simulink model "NUgus"  (R2018a)
settings: Solver=VariableStepAuto  StartTime=0.0  StopTime=inf  RelTol=1e-2
values from neighbouring files (symbols this model uses):
  CM740_acc_bias = 4 * 9.80743    (= 39.22972)    [CM740_init.m]
  CM740_acc_gain = 512 / CM740_acc_centre    [CM740_init.m]
  CM740_gyro_bias = 1600 / 360 * 2 * pi    (= 27.9252680319)    [CM740_init.m]
  CM740_gyro_gain = 512 / CM740_gyro_centre    [CM740_init.m]
  g = 9.8107    [init.m]
  head = [-0.05482228998067195, -0.00010888238321339966, 0.0011712900228573724, 0.41900000000000004]    [comtest.m]
  Kw = 0.9    [init.m]
  model = NUgusKinematics()    [KinematicsTest.m]    (also in Support_Region.m; init.m = NUgusKinematics)
  period = 1.0    (= 1)    [init.m]
  s = mean(abs(present_speed.data))    [RunServoTest.m]
  sample_time = 1/90    (= 0.0111111111111)    [init.m]
  step_height = 0.1    [init.m]
  torso = [0.0050079703254699804, 0.008880921777563762, 0.1021503146237477, 2.5390000000000006]    [comtest.m]
  z0 = 0.45    [init.m]
undefined symbols (not defined in the file or in its folder): sigbuilder_block, X, Y, Z
libraries: sm_lib x206, nesl_utility x82, Contact_Forces_Lib x10
(part 1 of 7)
settings Model: Creator=matt  LastModifiedBy=matt
settings SolverCC: MaxConsecutiveZCs=100  MinimalZcImpactIntegration=on
settings DebuggingCC: UniqueDataStoreMsg=error
settings ModelReferenceCC: ParallelModelReferenceMATLABWorkerInit=Copy Base Workspace  ModelReferenceNumInstancesAllowed=Single  ModelReferenceMinAlgLoopOccurrences=on
settings DiagnosticsConfigSet: SimMechanicsRigidlyBoundBlock=warning
settings ExplorerConfigSet: InternalSimMechanicsExplorerSettings="<ExplorerConfiguration><canonicalview>default</canonicalview><AnimationSetting><BasePlaybackSpeed>1.0</BasePlaybackSpeed><PlaybackSpeedFactor>0.125</PlaybackSpeedFactor></AnimationSetting><TilePanel><TileInfo><Tiles Columns=\"1\" Count=\"1\" Rows=\"1\"><Column Weight=\"1\"/><Row Weight=\"1\"/><Tile Height=\"1\" Width=\"1\" X=\"0\" Y=\"0\"/></Tiles></TileInfo><SceneInfo><SceneViewer><BGColor><R>0.800000011920928955</R><G>0.800000011920928955</G><B>0.800000011920928955</B></BGColor><Camera><DoPerspective>off</DoPerspective><Position><X>0.996097398048217064</X><Y>-0.871904325438711214</Y><Z>0.621451067428618886</Z></Position><Center><X>-0.122665475521987533</X><Y>0.224636309977359006</Y><Z>0.297935636755597033</Z></Center><Up><X>-0.160360573572373266</X><Y>0.125250173842771817</Y><Z>0.97907960881426559</Z></Up><ViewLimDist>1</ViewLimDist><YLim>0.594254607494361209</YLim><XLim>0.353738210919678941</XLim></Camera></SceneViewer></SceneInfo></TilePanel><MechEditorPanel><Cameras/><GfxPanelCameraMap/><VideoCreator><PlaybackSpeedRatio>1.0</PlaybackSpeedRatio><FrameRate>30</FrameRate><VideoFormat>Motion JPEG AVI</VideoFormat><FrameSize>auto</FrameSize></VideoCreator></MechEditorPanel></ExplorerConfiguration>"

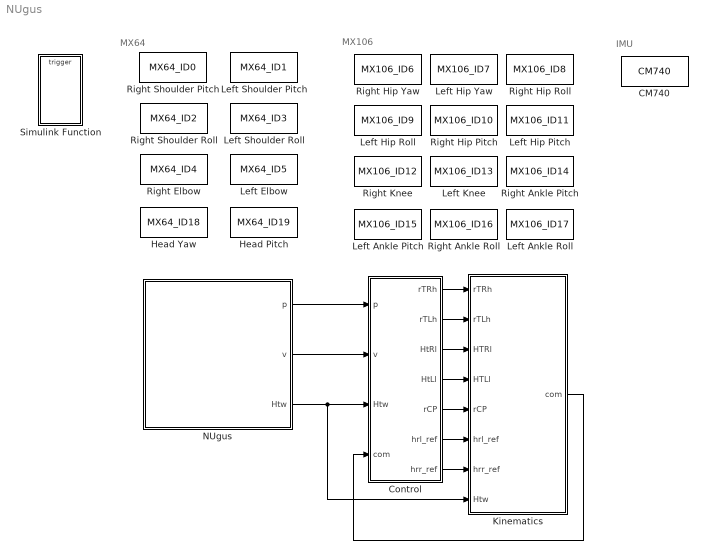
== system NUgus ==
  note: IMU
  note: MX64
  note: MX106
  CM740 : DataStoreMemory  DataStoreName=CM740  ReadBeforeWriteMsg=warning  WriteAfterWriteMsg=warning  WriteAfterReadMsg=warning  InitialValue=CM740_default  VectorParams1D=off  ShowAdditionalParam=off  OutDataTypeStr=Bus: CM740_bus
  Control : Subsystem
  Head Pitch : DataStoreMemory  DataStoreName=MX64_ID19  ReadBeforeWriteMsg=warning  WriteAfterWriteMsg=warning  WriteAfterReadMsg=warning  InitialValue=MX64_default  VectorParams1D=off  ShowAdditionalParam=off  OutDataTypeStr=Bus: MX64_bus
  Head Yaw : DataStoreMemory  DataStoreName=MX64_ID18  ReadBeforeWriteMsg=warning  WriteAfterWriteMsg=warning  WriteAfterReadMsg=warning  InitialValue=MX64_default  VectorParams1D=off  ShowAdditionalParam=off  OutDataTypeStr=Bus: MX64_bus
  Kinematics : Subsystem
  Left Ankle Pitch : DataStoreMemory  DataStoreName=MX106_ID15  ReadBeforeWriteMsg=warning  WriteAfterWriteMsg=warning  WriteAfterReadMsg=warning  InitialValue=MX106_default  VectorParams1D=off  ShowAdditionalParam=off  OutDataTypeStr=Bus: MX106_bus
  Left Ankle Roll : DataStoreMemory  DataStoreName=MX106_ID17  ReadBeforeWriteMsg=warning  WriteAfterWriteMsg=warning  WriteAfterReadMsg=warning  InitialValue=MX106_default  VectorParams1D=off  ShowAdditionalParam=off  OutDataTypeStr=Bus: MX106_bus
  Left Elbow : DataStoreMemory  DataStoreName=MX64_ID5  ReadBeforeWriteMsg=warning  WriteAfterWriteMsg=warning  WriteAfterReadMsg=warning  InitialValue=MX64_default  VectorParams1D=off  ShowAdditionalParam=off  OutDataTypeStr=Bus: MX64_bus
  Left Hip Pitch : DataStoreMemory  DataStoreName=MX106_ID11  ReadBeforeWriteMsg=warning  WriteAfterWriteMsg=warning  WriteAfterReadMsg=warning  InitialValue=MX106_default  VectorParams1D=off  ShowAdditionalParam=off  OutDataTypeStr=Bus: MX106_bus
  Left Hip Roll : DataStoreMemory  DataStoreName=MX106_ID9  ReadBeforeWriteMsg=warning  WriteAfterWriteMsg=warning  WriteAfterReadMsg=warning  InitialValue=MX106_default  VectorParams1D=off  ShowAdditionalParam=off  OutDataTypeStr=Bus: MX106_bus
  Left Hip Yaw : DataStoreMemory  DataStoreName=MX106_ID7  ReadBeforeWriteMsg=warning  WriteAfterWriteMsg=warning  WriteAfterReadMsg=warning  InitialValue=MX106_default  VectorParams1D=off  ShowAdditionalParam=off  OutDataTypeStr=Bus: MX106_bus
  Left Knee : DataStoreMemory  DataStoreName=MX106_ID13  ReadBeforeWriteMsg=warning  WriteAfterWriteMsg=warning  WriteAfterReadMsg=warning  InitialValue=MX106_default  VectorParams1D=off  ShowAdditionalParam=off  OutDataTypeStr=Bus: MX106_bus
  Left Shoulder Pitch : DataStoreMemory  DataStoreName=MX64_ID1  ReadBeforeWriteMsg=warning  WriteAfterWriteMsg=warning  WriteAfterReadMsg=warning  InitialValue=MX64_default  VectorParams1D=off  ShowAdditionalParam=off  OutDataTypeStr=Bus: MX64_bus
  Left Shoulder Roll : DataStoreMemory  DataStoreName=MX64_ID3  ReadBeforeWriteMsg=warning  WriteAfterWriteMsg=warning  WriteAfterReadMsg=warning  InitialValue=MX64_default  VectorParams1D=off  ShowAdditionalParam=off  OutDataTypeStr=Bus: MX64_bus
  NUgus : Subsystem
      mask Display: image('./img/NUgus.png');
  Right Ankle Pitch : DataStoreMemory  DataStoreName=MX106_ID14  ReadBeforeWriteMsg=warning  WriteAfterWriteMsg=warning  WriteAfterReadMsg=warning  InitialValue=MX106_default  VectorParams1D=off  ShowAdditionalParam=off  OutDataTypeStr=Bus: MX106_bus
  Right Ankle Roll : DataStoreMemory  DataStoreName=MX106_ID16  ReadBeforeWriteMsg=warning  WriteAfterWriteMsg=warning  WriteAfterReadMsg=warning  InitialValue=MX106_default  VectorParams1D=off  ShowAdditionalParam=off  OutDataTypeStr=Bus: MX106_bus
  Right Elbow : DataStoreMemory  DataStoreName=MX64_ID4  ReadBeforeWriteMsg=warning  WriteAfterWriteMsg=warning  WriteAfterReadMsg=warning  InitialValue=MX64_default  VectorParams1D=off  ShowAdditionalParam=off  OutDataTypeStr=Bus: MX64_bus
  Right Hip Pitch : DataStoreMemory  DataStoreName=MX106_ID10  ReadBeforeWriteMsg=warning  WriteAfterWriteMsg=warning  WriteAfterReadMsg=warning  InitialValue=MX106_default  VectorParams1D=off  ShowAdditionalParam=off  OutDataTypeStr=Bus: MX106_bus
  Right Hip Roll : DataStoreMemory  DataStoreName=MX106_ID8  ReadBeforeWriteMsg=warning  WriteAfterWriteMsg=warning  WriteAfterReadMsg=warning  InitialValue=MX106_default  VectorParams1D=off  ShowAdditionalParam=off  OutDataTypeStr=Bus: MX106_bus
  Right Hip Yaw : DataStoreMemory  DataStoreName=MX106_ID6  InitialValue=MX106_default  VectorParams1D=off  ShowAdditionalParam=off  OutDataTypeStr=Bus: MX106_bus
  Right Knee : DataStoreMemory  DataStoreName=MX106_ID12  ReadBeforeWriteMsg=warning  WriteAfterWriteMsg=warning  WriteAfterReadMsg=warning  InitialValue=MX106_default  VectorParams1D=off  ShowAdditionalParam=off  OutDataTypeStr=Bus: MX106_bus
  Right Shoulder Pitch : DataStoreMemory  DataStoreName=MX64_ID0  ReadBeforeWriteMsg=warning  WriteAfterWriteMsg=warning  WriteAfterReadMsg=warning  InitialValue=MX64_default  VectorParams1D=off  ShowAdditionalParam=off  OutDataTypeStr=Bus: MX64_bus
  Right Shoulder Roll : DataStoreMemory  DataStoreName=MX64_ID2  ReadBeforeWriteMsg=warning  WriteAfterWriteMsg=warning  WriteAfterReadMsg=warning  InitialValue=MX64_default  VectorParams1D=off  ShowAdditionalParam=off  OutDataTypeStr=Bus: MX64_bus
  Simulink Function : Subsystem  TreatAsAtomicUnit=on
  wires:
  NUgus/1(p) -> Control/1(p)
  NUgus/2(v) -> Control/2(v)
  Control/1(rTRh) -> Kinematics/1(rTRh)
  Control/2(rTLh) -> Kinematics/2(rTLh)
  Control/3(HtRl) -> Kinematics/3(HTRl)
  Control/4(HtLl) -> Kinematics/4(HTLl)
  Control/5(rCP) -> Kinematics/5(rCP)
  NUgus/3(Htw) -> Control/3(Htw), Kinematics/8(Htw)
  Kinematics/1(com) -> Control/4(com)
  Control/6(hrl_ref) -> Kinematics/6(hrl_ref)
  Control/7(hrr_ref) -> Kinematics/7(hrr_ref)

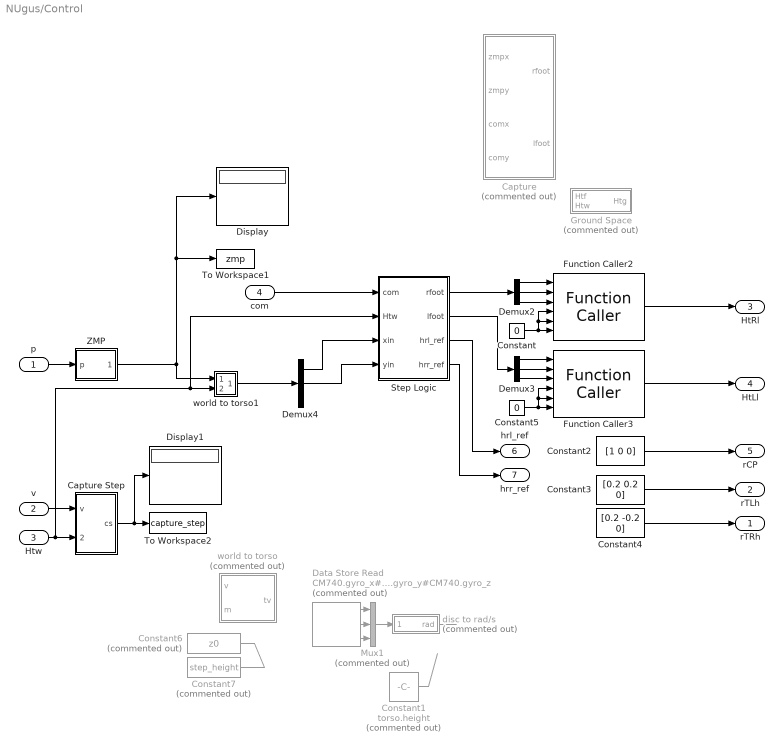
== system NUgus/Control ==
  p : Inport
  v : Inport  Port=2
  Htw : Inport  Port=3
  com : Inport  Port=4
  Capture : Stateflow chart  Commented=on  TreatAsAtomicUnit=on
  Capture Step : Subsystem
  Constant : Constant  Value=0
  Constant1 : Constant  Commented=on  Value=torso.height
  Constant2 : Constant  Value=[1 0 0]
  Constant3 : Constant  Value=[0.2 0.2 0]
  Constant4 : Constant  Value=[0.2 -0.2 0]
  Constant5 : Constant  Value=0
  Constant6 : Constant  Commented=on  Value=z0
  Constant7 : Constant  Commented=on  Value=step_height
  Data Store Read : DataStoreRead  Commented=on  DataStoreName=CM740  SampleTime=1/90  DataStoreElements=CM740.gyro_x#CM740.gyro_y#CM740.gyro_z
  Demux2 : Demux  Outputs=3
  Demux3 : Demux  Outputs=3
  Demux4 : Demux  Outputs=3
  Display : Display
  Display1 : Display
  Function Caller2 : FunctionCaller  FunctionPrototype=H = getTransform(x,y,z,roll,pitch,yaw)
  Function Caller3 : FunctionCaller  FunctionPrototype=H = getTransform(x,y,z,roll,pitch,yaw)
  Ground Space : MATLAB Function  Commented=on  TreatAsAtomicUnit=on
  Mux1 : Mux  Commented=on  Inputs=3
  Step Logic : Stateflow chart  TreatAsAtomicUnit=on
  To Workspace1 : ToWorkspace  VariableName=zmp  SaveFormat=Timeseries  SampleTime=sample_time
  To Workspace2 : ToWorkspace  VariableName=capture_step  SaveFormat=Timeseries  SampleTime=sample_time
  ZMP : Subsystem
  disc to rad/s : Subsystem  Commented=on
  world to torso : Subsystem  Commented=on
  world to torso1 : Subsystem
  rTRh : Outport
  rTLh : Outport  Port=2
  HtRl : Outport  Port=3
  HtLl : Outport  Port=4
  rCP : Outport  Port=5
  hrl_ref : Outport  Port=6
  hrr_ref : Outport  Port=7
  wires:
  Demux2/3 -> Function Caller2/3
  Demux3/3 -> Function Caller3/3
  disc to rad/s/1(rad) -> ?
  Demux3/2 -> Function Caller3/2
  Constant/1 -> Function Caller2/4, Function Caller2/5, Function Caller2/6
  Data Store Read/3 -> Mux1/3
  Step Logic/1(rfoot) -> Demux2/1
  Data Store Read/2 -> Mux1/2
  Mux1/1 -> disc to rad/s/1(disc)
  Demux2/2 -> Function Caller2/2
  Data Store Read/1 -> Mux1/1
  Demux3/1 -> Function Caller3/1
  Demux2/1 -> Function Caller2/1
  Step Logic/2(lfoot) -> Demux3/1
  p/1 -> ZMP/1(p)
  Htw/1 -> Step Logic/2(Htw), world to torso1/2(m), Capture Step/2(Htw)
  Capture Step/1(cs) -> Display1/1, To Workspace2/1
  v/1 -> Capture Step/1(v)
  Constant1/1 -> ?
  Constant2/1 -> rCP/1
  Constant3/1 -> rTLh/1
  Constant4/1 -> rTRh/1
  Constant5/1 -> Function Caller3/4, Function Caller3/5, Function Caller3/6
  Constant6/1 -> ?
  Constant7/1 -> ?
  ZMP/1(zmp) -> world to torso1/1(v), To Workspace1/1, Display/1
  Function Caller3/1 -> HtLl/1
  Function Caller2/1 -> HtRl/1
  Step Logic/3(hrl_ref) -> hrl_ref/1
  Step Logic/4(hrr_ref) -> hrr_ref/1
  Demux4/2 -> Step Logic/4(yin)
  Demux4/1 -> Step Logic/3(xin)
  com/1 -> Step Logic/1(com)
  world to torso1/1(tv) -> Demux4/1

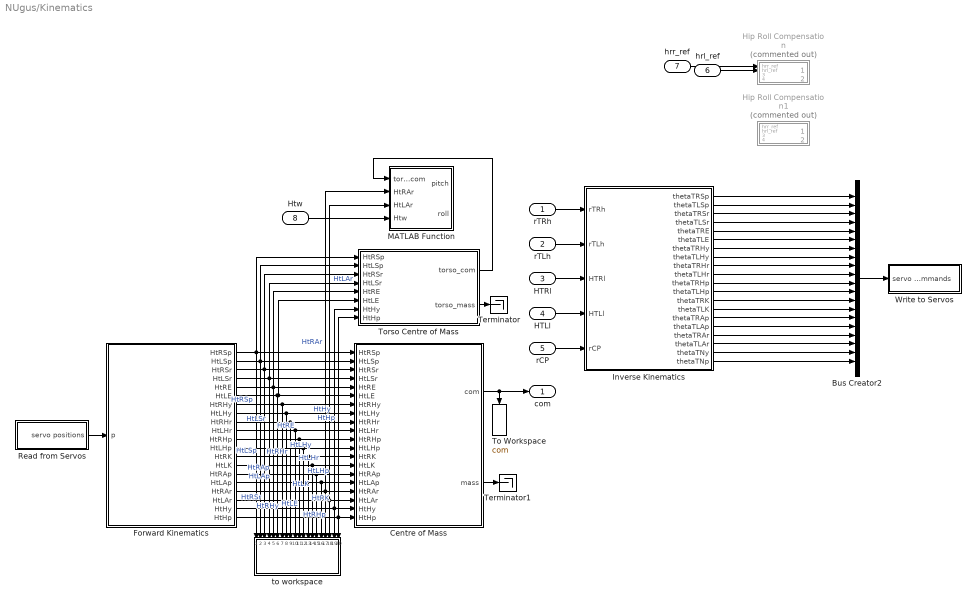
== system NUgus/Kinematics ==
  rTRh : Inport
  rTLh : Inport  Port=2
  HTRl : Inport  Port=3
  HTLl : Inport  Port=4
  rCP : Inport  Port=5
  hrl_ref : Inport  Port=6
  hrr_ref : Inport  Port=7
  Htw : Inport  Port=8
  Bus Creator2 : BusCreator  Inputs=20
  Centre of Mass : Subsystem
  Forward Kinematics : Subsystem
  Hip Roll Compensation : Subsystem  Commented=on
  Hip Roll Compensation1 : Subsystem  Commented=on
  Inverse Kinematics : Subsystem
  MATLAB Function : MATLAB Function  TreatAsAtomicUnit=on  SystemSampleTime=sample_time
  Read from Servos : Subsystem
  Terminator : Terminator
  Terminator1 : Terminator
  To Workspace : ToWorkspace  VariableName=com  SaveFormat=Timeseries  SampleTime=sample_time
  Torso Centre of Mass : Subsystem
  Write to Servos : Subsystem
  to workspace : Subsystem
  com : Outport
  wires:
  Forward Kinematics/10(HtLHr) -> Centre of Mass/10(HtLHr), to workspace/10(HtLHr)  "HtLHr"
  Forward Kinematics/9(HtRHr) -> Centre of Mass/9(HtRHr), to workspace/9(HtRHr)  "HtRHr"
  Forward Kinematics/8(HtLHy) -> Centre of Mass/8(HtLHy), to workspace/8(HtLHy)  "HtLHy"
  Inverse Kinematics/19(thetaTNy) -> Bus Creator2/19
  Forward Kinematics/12(HtLHp) -> Centre of Mass/12(HtLHp), to workspace/12(HtLHp)  "HtLHp"
  Forward Kinematics/15(HtRAp) -> Centre of Mass/15(HtRAp), to workspace/15(HtRAp)  "HtRAp"
  Centre of Mass/1(com) -> com/1, To Workspace/1
  HTLl/1 -> Inverse Kinematics/4(HTLl)
  Forward Kinematics/11(HtRHp) -> Centre of Mass/11(HtRHp), to workspace/11(HtRHp)  "HtRHp"
  Forward Kinematics/4(HtLSr) -> Torso Centre of Mass/4(HtLSr), Centre of Mass/4(HtLSr), to workspace/4(HtLSr)  "HtLSr"
  Inverse Kinematics/5(thetaTRE) -> Bus Creator2/5
  Forward Kinematics/18(HtLAr) -> Centre of Mass/18(HtLAr), MATLAB Function/3(HtLAr), to workspace/18(HtLAr)  "HtLAr"
  rTRh/1 -> Inverse Kinematics/1(rTRh)
  Inverse Kinematics/6(thetaTLE) -> Bus Creator2/6
  Forward Kinematics/6(HtLE) -> Torso Centre of Mass/6(HtLE), Centre of Mass/6(HtLE), to workspace/6(HtLE)  "HtLE"
  Forward Kinematics/14(HtLK) -> Centre of Mass/14(HtLK), to workspace/14(HtLK)  "HtLK"
  Forward Kinematics/13(HtRK) -> Centre of Mass/13(HtRK), to workspace/13(HtRK)  "HtRK"
  Forward Kinematics/3(HtRSr) -> Torso Centre of Mass/3(HtRSr), Centre of Mass/3(HtRSr), to workspace/3(HtRSr)  "HtRSr"
  Inverse Kinematics/14(thetaTLK) -> Bus Creator2/14
  Inverse Kinematics/7(thetaTRHy) -> Bus Creator2/7
  Forward Kinematics/2(HtLSp) -> Torso Centre of Mass/2(HtLSp), Centre of Mass/2(HtLSp), to workspace/2(HtLSp)  "HtLSp"
  Forward Kinematics/7(HtRHy) -> Centre of Mass/7(HtRHy), to workspace/7(HtRHy)  "HtRHy"
  Forward Kinematics/5(HtRE) -> Torso Centre of Mass/5(HtRE), Centre of Mass/5(HtRE), to workspace/5(HtRE)  "HtRE"
  Forward Kinematics/20(HtHp) -> to workspace/20(HtHp), Torso Centre of Mass/8(HtHp), Centre of Mass/20(HtHp)  "HtHp"
  Inverse Kinematics/1(thetaTRSp) -> Bus Creator2/1
  Inverse Kinematics/3(thetaTRSr) -> Bus Creator2/3
  Inverse Kinematics/13(thetaTRK) -> Bus Creator2/13
  Forward Kinematics/16(HtLAp) -> Centre of Mass/16(HtLAp), to workspace/16(HtLAp)  "HtLAp"
  Forward Kinematics/19(HtHy) -> to workspace/19(HtHy), Torso Centre of Mass/7(HtHy), Centre of Mass/19(HtHy)  "HtHy"
  Read from Servos/1(servo positions) -> Forward Kinematics/1(p)
  rTLh/1 -> Inverse Kinematics/2(rTLh)
  Bus Creator2/1 -> Write to Servos/1(servo commands)
  Forward Kinematics/1(HtRSp) -> Torso Centre of Mass/1(HtRSp), Centre of Mass/1(HtRSp), to workspace/1(HtRSp)  "HtRSp"
  Inverse Kinematics/2(thetaTLSp) -> Bus Creator2/2
  Inverse Kinematics/20(thetaTNp) -> Bus Creator2/20
  Inverse Kinematics/4(thetaTLSr) -> Bus Creator2/4
  Forward Kinematics/17(HtRAr) -> to workspace/17(HtRAr), MATLAB Function/2(HtRAr), Centre of Mass/17(HtRAr)  "HtRAr"
  HTRl/1 -> Inverse Kinematics/3(HTRl)
  rCP/1 -> Inverse Kinematics/5(rCP)
  Torso Centre of Mass/2(torso_mass) -> Terminator/1
  Htw/1 -> MATLAB Function/4(Htw)
  Torso Centre of Mass/1(torso_com) -> MATLAB Function/1(torso_com)
  Inverse Kinematics/16(thetaTLAp) -> Bus Creator2/16
  Inverse Kinematics/15(thetaTRAp) -> Bus Creator2/15
  Inverse Kinematics/11(thetaTRHp) -> Bus Creator2/11
  Inverse Kinematics/12(thetaTLHp) -> Bus Creator2/12
  Inverse Kinematics/17(thetaTRAr) -> Bus Creator2/17
  Inverse Kinematics/18(thetaTLAr) -> Bus Creator2/18
  Inverse Kinematics/8(thetaTLHy) -> Bus Creator2/8
  Centre of Mass/2(mass) -> Terminator1/1
  hrl_ref/1 -> Hip Roll Compensation/2(hrl_ref)
  hrr_ref/1 -> Hip Roll Compensation/1("hrr_ref ")
  Inverse Kinematics/9(thetaTRHr) -> Bus Creator2/9
  Inverse Kinematics/10(thetaTLHr) -> Bus Creator2/10

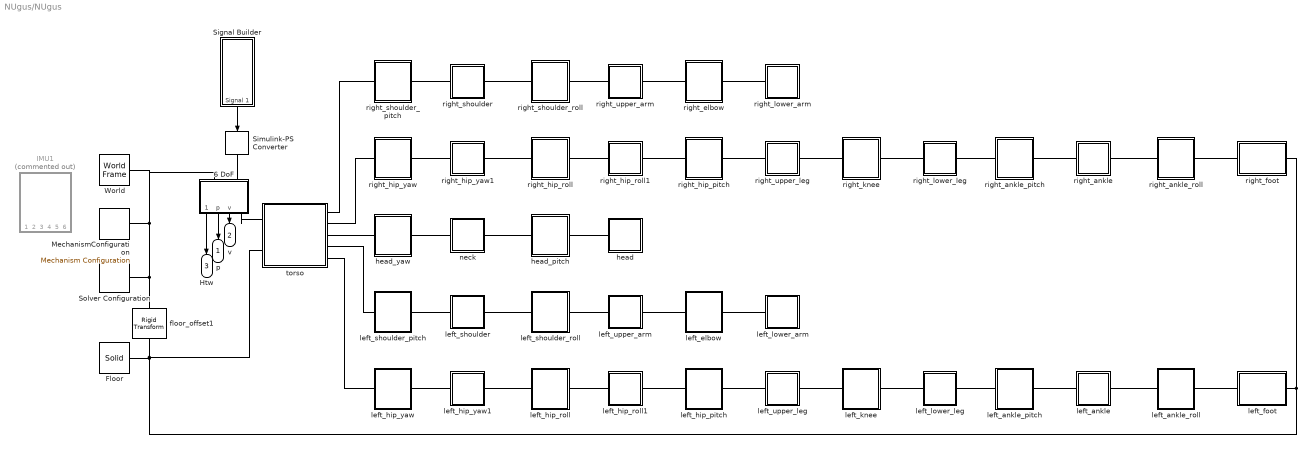
== system NUgus/NUgus ==
  6 DoF : Subsystem
  Floor : sm_lib/Body Elements/Solid  InertiaType=CalculateFromGeometry  Mass=1  MassUnits=kg  CenterOfMass=[0 0 0]  CenterOfMassUnits=m  MomentsOfInertia=[1 1 1]  MomentsOfInertiaUnits=kg*m^2  ProductsOfInertia=[0 0 0]  ProductsOfInertiaUnits=kg*m^2  DensityBased=on  Density=1000  DensityUnits=kg/m^3  DoExposeReferenceFrame=on  SerializedFrames=<Frames/>  GraphicType=FromGeometry  MarkerShape=Frame  MarkerSize=10  GraphicVisPropType=SimpleVisualProperties  GraphicDiffuseColor=[0.972549 0.972549 0.972549]  GraphicSpecularColor=[0.3 0.3 0.3 1.0]  GraphicAmbientColor=[0.20 0.20 0.20 1.0]  GraphicEmissiveColor=[0.0 0.0 0.0 1.0]  GraphicShininess=30  GraphicOpacity=0.6  GeometryShape=Brick  RectangleSize=[1 1]  RectangleSizeUnits=m  BrickDimensions=[floor.length floor.width floor.depth]  BrickDimensionUnits=m  CylinderRadius=1  CylinderRadiusUnits=m  CylinderLength=1  CylinderLengthUnits=m  SphereRadius=1  SphereRadiusUnits=m  EllipsoidRadii=[1 1 1]  EllipsoidRadiiUnits=m  ExtrusionCrossSection=[1 1; -1 1; -1 -1; 1 -1]  ExtrusionCrossSectionUnits=m  ExtrusionLength=1  ExtrusionLengthUnits=m  PolygonNumSides=3  PolygonOuterRadius=1  PolygonOuterRadiusUnits=m  ExtGeomFileType=STEP  ExtGeomFileUnits=m  RevolutionCrossSection=[1 1; 1 -1; 2 -1; 2 1]  RevolutionCrossSectionUnits=m  RevolutionExtent=Full  RevolutionAngle=180  RevolutionAngleUnits=deg
  IMU1 : Subsystem  Commented=on
  MechanismConfiguration : sm_lib/Utilities/Mechanism Configuration  UniformGravity=Constant  GravityVector=[0 0 -9.80665]  GravityUnits=m/s^2  LinearizationDelta=0.001
  Signal Builder : Subsystem  Tag=STV Subsys  LoadFcn=sigbuilder_block('load');  StartFcn=sigbuilder_block('start');  StopFcn=sigbuilder_block('stop');  ClipboardFcn=sigbuilder_block('clipboard');  mask(Sigbuilder block){tuvar=[0:10]}
      mask help: Simulink:masks:SigbuilderBlock_MD
      mask init:
      | if ~strcmp(get_param(bdroot(gcbh),'SimulationStatus'),'stopped') tuvar = sigbuilder_block('maskInit'); end
      settings: CopyFcn=sigbuilder_block('copy');  DeleteFcn=sigbuilder_block('delete');  ModelCloseFcn=sigbuilder_block('modelClose');  PreSaveFcn=sigbuilder_block('preSave');  PauseFcn=sigbuilder_block('pause');  ContinueFcn=sigbuilder_block('continue');  NameChangeFcn=sigbuilder_block('namechange');  OpenFcn=sigbuilder_block('open',[1006.5 174.75 565.5 399.75 ]);  CloseFcn=sigbuilder_block('close');
      mask Display: plot(0, 0, 100, 100,[2, 2, 32, 32, 2], [68, 8, 8, 68, 68],[32, 2], [38, 38], [32, 19, 2],[53, 60, 44], [32, 17, 17, 2],[16, 16, 31, 31]);txt = getActiveGroup(gcbh);text(2, 100, txt,'verticalAlignment', 'top');
  Simulink-PS Converter : nesl_utility/Simulink-PS Converter  PhysicalDomain=network_engine_domain  SubClassName=ps_input  LeftPortType=input  RightPortType=output  PseudoPeriodic=off  Frequencies=[]  NoiseDistribution=none  NoiseParameters=[]  Unit=N  AffineConversion=off  FilteringAndDerivatives=provide  SimscapeFilterOrder=1  InputFilterTimeConstant=0.001  UdotUserProvided=0
  Solver Configuration : nesl_utility/Solver Configuration  PhysicalDomain=network_engine_domain  SubClassName=solver  LeftPortType=input  RightPortType=generic  Tones=[]  Harmonics=[]  SimulateNoise=off  Profile=off  UseLocalSampling=off  EnableSwitchedLinearOptims=on  FrequencyDomain=off  UseCCode=off  RelTol=0.001  AbsTol=1e-06  MinStep=1e-09  ToWorkspace=off  RevertToSquareIcSolve=off  NumHomotopyIterations=100  PhasorMode=off  PhasorModeNumHarmonics=1  DoDC=off  ResidualTolerance=1e-03  UseLocalSolver=off  LocalSolverChoice=NE_BACKWARD_EULER_ADVANCER  LocalSolverSampleTime=0.001  DoFixedCost=off  MaxNonlinIter=3  MaxModeIter=2  LinearAlgebra=Sparse  EquationFormulation=NE_TIME_EF  DelaysMemoryBudget=1024  AutomaticFiltering=on  FilteringTimeConstant=0.001
  World : sm_lib/Frames and Transforms/World Frame
  floor_offset1 : sm_lib/Frames and Transforms/Rigid Transform  TranslationMethod=Cartesian  TranslationStandardOffset=0  TranslationLengthUnit=m  TranslationStandardAxis=+Z  TranslationCartesianOffset=[0 0 -floor.depth/2]  TranslationROffset=0  TranslationROffsetUnits=m  TranslationZOffset=0  TranslationZOffsetUnits=m  TranslationThetaOffset=0  TranslationThetaOffsetUnits=deg  RotationMethod=None  RotationAngleUnits=deg  RotationStandardAxis=+Z  RotationAngle=0.0  RotationArbitraryAxis=[0 0 1]  FollAlignAxisA=+X  BaseAlignAxisA=+Y  FollAlignAxisB=+Y  BaseAlignAxisB=+Z  RotationSequenceAxes=FollowerAxes  RotationSequence=XYX  RotationSequenceAngles=[0 0 0]  RotationSequenceAnglesUnits=deg  RotationMatrix=[1 0 0; 0 1 0; 0 0 1]
  head : Subsystem
  head_pitch : Subsystem
      mask Display: image('./img/MX64.png');
  head_yaw : Subsystem
      mask Display: image('./img/MX64.png');
  left_ankle : Subsystem
  left_ankle_pitch : Subsystem
      mask Display: image('./img/MX106.png');
  left_ankle_roll : Subsystem
      mask Display: image('./img/MX106.png');
  left_elbow : Subsystem
      mask Display: image('./img/MX64.png');
  left_foot : Subsystem
  left_hip_pitch : Subsystem
      mask Display: image('./img/MX106.png');
  left_hip_roll : Subsystem
      mask Display: image('./img/MX106.png');
  left_hip_roll1 : Subsystem
  left_hip_yaw : Subsystem
      mask Display: image('./img/MX106.png');
  left_hip_yaw1 : Subsystem
  left_knee : Subsystem
      mask Display: image('./img/MX106.png');
  left_lower_arm : Subsystem
  left_lower_leg : Subsystem
  left_shoulder : Subsystem
  left_shoulder_pitch : Subsystem
      mask Display: image('./img/MX64.png');
  left_shoulder_roll : Subsystem
      mask Display: image('./img/MX64.png');
  left_upper_arm : Subsystem
  left_upper_leg : Subsystem
  neck : Subsystem
  right_ankle : Subsystem
  right_ankle_pitch : Subsystem
      mask Display: image('./img/MX106.png');
  right_ankle_roll : Subsystem
      mask Display: image('./img/MX106.png');
  right_elbow : Subsystem
      mask Display: image('./img/MX64.png');
  right_foot : Subsystem
  right_hip_pitch : Subsystem
      mask Display: image('./img/MX106.png');
  right_hip_roll : Subsystem
      mask Display: image('./img/MX106.png');
  right_hip_roll1 : Subsystem
  right_hip_yaw : Subsystem
      mask Display: image('./img/MX106.png');
  right_hip_yaw1 : Subsystem
  right_knee : Subsystem
      mask Display: image('./img/MX106.png');
  right_lower_arm : Subsystem
  right_lower_leg : Subsystem
  right_shoulder : Subsystem
  right_shoulder_pitch : Subsystem
      mask Display: image('./img/MX64.png');
  right_shoulder_roll : Subsystem
      mask Display: image('./img/MX64.png');
  right_upper_arm : Subsystem
  right_upper_leg : Subsystem
  torso : Subsystem
  p : Outport
  v : Outport  Port=2
  Htw : Outport  Port=3
  wires:
  Signal Builder/1(Signal 1) -> Simulink-PS Converter/1
  6 DoF/2(p) -> p/1
  6 DoF/3(v) -> v/1
  6 DoF/1(Htw) -> Htw/1
  connections:
  right_ankle_roll/LConn1 -- right_ankle/RConn1
  left_elbow/RConn1 -- left_lower_arm/LConn1
  left_knee/RConn1 -- left_lower_leg/LConn1
  left_hip_roll/LConn1 -- left_hip_yaw1/RConn1
  left_hip_yaw/RConn1 -- left_hip_yaw1/LConn1
  torso/RConn3 -- head_yaw/LConn1
  right_shoulder_roll/LConn1 -- right_shoulder/RConn1
  right_hip_pitch/LConn1 -- right_hip_roll1/RConn1
  right_hip_yaw1/RConn1 -- right_hip_roll/LConn1
  head_pitch/LConn1 -- neck/RConn1
  right_lower_arm/LConn1 -- right_elbow/RConn1
  head/LConn1 -- head_pitch/RConn1
  left_shoulder/RConn1 -- left_shoulder_roll/LConn1
  left_hip_pitch/RConn1 -- left_upper_leg/LConn1
  left_foot/LConn1 -- left_ankle_roll/RConn1
  torso/RConn1 -- right_shoulder_pitch/LConn1
  right_hip_pitch/RConn1 -- right_upper_leg/LConn1
  right_hip_yaw/LConn1 -- torso/RConn2
  left_shoulder_pitch/LConn1 -- torso/RConn4
  left_ankle_pitch/RConn1 -- left_ankle/LConn1
  left_ankle_pitch/LConn1 -- left_lower_leg/RConn1
  left_knee/LConn1 -- left_upper_leg/RConn1
  left_hip_roll/RConn1 -- left_hip_roll1/LConn1
  left_upper_arm/LConn1 -- left_shoulder_roll/RConn1
  left_shoulder_pitch/RConn1 -- left_shoulder/LConn1
  left_ankle_roll/LConn1 -- left_ankle/RConn1
  right_ankle_pitch/RConn1 -- right_ankle/LConn1
  right_ankle_pitch/LConn1 -- right_lower_leg/RConn1
  neck/LConn1 -- head_yaw/RConn1
  right_knee/RConn1 -- right_lower_leg/LConn1
  right_ankle_roll/RConn1 -- right_foot/LConn1
  right_knee/LConn1 -- right_upper_leg/RConn1
  right_hip_roll1/LConn1 -- right_hip_roll/RConn1
  right_shoulder_pitch/RConn1 -- right_shoulder/LConn1
  right_elbow/LConn1 -- right_upper_arm/RConn1
  right_hip_yaw/RConn1 -- right_hip_yaw1/LConn1
  left_elbow/LConn1 -- left_upper_arm/RConn1
  left_hip_roll1/RConn1 -- left_hip_pitch/LConn1
  torso/RConn5 -- left_hip_yaw/LConn1
  right_shoulder_roll/RConn1 -- right_upper_arm/LConn1
  left_foot/RConn1 -- torso/LConn2 -- floor_offset1/RConn1 -- Floor/RConn1 -- right_foot/RConn1
  6 DoF/RConn1 -- torso/LConn1
  MechanismConfiguration/RConn1 -- 6 DoF/LConn1 -- World/RConn1 -- floor_offset1/LConn1 -- Solver Configuration/RConn1
  Simulink-PS Converter/RConn1 -- 6 DoF/LConn2

== system NUgus/Simulink Function ==
  getTransform : TriggerPort  TriggerType=function-call  IsSimulinkFunction=on  FunctionName=getTransform  FunctionVisibility=scoped  VariantControl=(inherit)
  MATLAB Function : MATLAB Function  TreatAsAtomicUnit=on
  x : ArgIn  DisableCoverage=on  ArgumentName=x
  y~ : ArgIn  Port=2  ArgumentName=y
  z : ArgIn  Port=3  ArgumentName=z
  roll : ArgIn  Port=4  ArgumentName=roll
  pitch : ArgIn  Port=5  ArgumentName=pitch
  yaw : ArgIn  Port=6  ArgumentName=yaw
  H : ArgOut  DisableCoverage=on  PortDimensions=[4 4]  ArgumentName=H
  wires:
  x/1 -> MATLAB Function/1(x)
  y~/1 -> MATLAB Function/2(y)
  z/1 -> MATLAB Function/3(z)
  roll/1 -> MATLAB Function/4(roll)
  pitch/1 -> MATLAB Function/5(pitch)
  yaw/1 -> MATLAB Function/6(yaw)
  MATLAB Function/1(H) -> H/1

== system NUgus/Control/Capture Step ==
  v : Inport
  Htw : Inport  Port=2
  Gain : Gain  Gain=sqrt(torso.height/g)
  Matrix Multiply : Product  Multiplication=Matrix(*)
  Subsystem3 : Subsystem
  Subsystem4 : Subsystem
  cs : Outport
  wires:
  Matrix Multiply/1 -> Subsystem4/1(v4)
  Gain/1 -> Subsystem3/1(v3)
  Subsystem4/1(v3) -> cs/1
  v/1 -> Gain/1
  Subsystem3/1(v4) -> Matrix Multiply/2
  Htw/1 -> Matrix Multiply/1

== system NUgus/Control/ZMP ==
  note: zmp z = 0
  note: h = p com,z / g
  note: zmp = p com - ha com
  note: 3D LIPM ZMP Model
  p : Inport
  Add : Sum  Inputs=-+
  Data Store Read : DataStoreRead  DataStoreName=CM740  SampleTime=1/90  DataStoreElements=CM740.acc_x#CM740.acc_y#CM740.acc_z
  Demux : Demux  Outputs=3
  Multiply1 : Product
  Mux : Mux  Inputs=3
  Mux2 : Mux  Inputs=3
  h : Gain  Gain=1/g
  to real : Subsystem
  zmp : Outport
  wires:
  p/1 -> Demux/1
  to real/1(continuous) -> Multiply1/1
  Add/1 -> zmp/1
  Multiply1/1 -> Add/1
  h/1 -> Multiply1/2
  Demux/3 -> Mux2/3, h/1
  Demux/2 -> Mux2/2
  Demux/1 -> Mux2/1
  Mux2/1 -> Add/2
  Data Store Read/2 -> Mux/2
  Data Store Read/1 -> Mux/1
  Data Store Read/3 -> Mux/3
  Mux/1 -> to real/1(discrete)

== system NUgus/Control/disc to rad//s ==
  disc : Inport
  Add1 : Sum  Inputs=+-
  Constant4 : Constant  Value=512
  Gain : Gain  Gain=(500*pi)/(180*512)  OutDataTypeStr=double
  rad : Outport
  wires:
  disc/1 -> Add1/1
  Gain/1 -> rad/1
  Add1/1 -> Gain/1
  Constant4/1 -> Add1/2

== system NUgus/Control/world to torso ==
  v : Inport
  m : Inport  Port=2
  Matrix Multiply : Product  Multiplication=Matrix(*)
  Subsystem3 : Subsystem
  Subsystem4 : Subsystem
  tv : Outport
  wires:
  v/1 -> Subsystem3/1(v3)
  Matrix Multiply/1 -> Subsystem4/1(v4)
  m/1 -> Matrix Multiply/1
  Subsystem4/1(v3) -> tv/1
  Subsystem3/1(v4) -> Matrix Multiply/2

== system NUgus/Control/world to torso1 ==
  v : Inport
  m : Inport  Port=2
  Matrix Multiply : Product  Multiplication=Matrix(*)
  Subsystem3 : Subsystem
  Subsystem4 : Subsystem
  tv : Outport
  wires:
  v/1 -> Subsystem3/1(v3)
  Matrix Multiply/1 -> Subsystem4/1(v4)
  m/1 -> Matrix Multiply/1
  Subsystem4/1(v3) -> tv/1
  Subsystem3/1(v4) -> Matrix Multiply/2

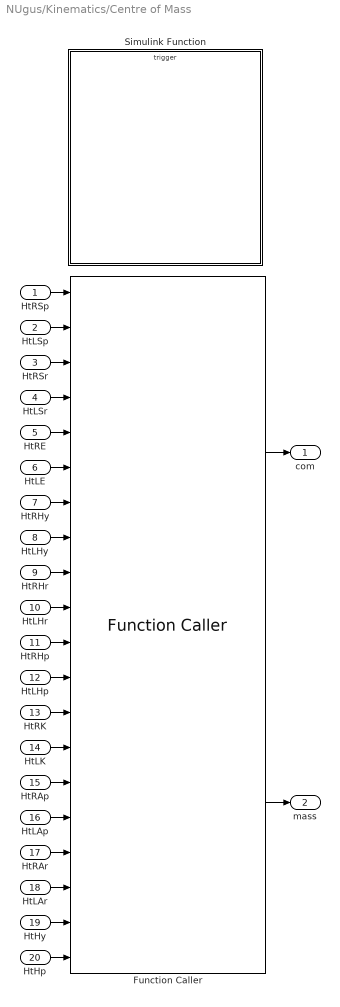
== system NUgus/Kinematics/Centre of Mass ==
  HtRSp : Inport
  HtLSp : Inport  Port=2
  HtRSr : Inport  Port=3
  HtLSr : Inport  Port=4
  HtRE : Inport  Port=5
  HtLE : Inport  Port=6
  HtRHy : Inport  Port=7
  HtLHy : Inport  Port=8
  HtRHr : Inport  Port=9
  HtLHr : Inport  Port=10
  HtRHp : Inport  Port=11
  HtLHp : Inport  Port=12
  HtRK : Inport  Port=13
  HtLK : Inport  Port=14
  HtRAp : Inport  Port=15
  HtLAp : Inport  Port=16
  HtRAr : Inport  Port=17
  HtLAr : Inport  Port=18
  HtHy : Inport  Port=19
  HtHp : Inport  Port=20
  Function Caller : FunctionCaller  FunctionPrototype=[com,mass] = COM(HtRSp,HtLSp,HtRSr,HtLSr,HtRE,HtLE,HtRHy,HtLHy,HtRHr,HtLHr,HtRHp,HtLHp,HtRK,HtLK,HtRAp,HtLAp,HtRAr,HtLAr,HtHy,HtHp)
  Simulink Function : Subsystem  TreatAsAtomicUnit=on
  com : Outport
  mass : Outport  Port=2
  wires:
  HtRK/1 -> Function Caller/13
  HtRHp/1 -> Function Caller/11
  HtHy/1 -> Function Caller/19
  HtLHp/1 -> Function Caller/12
  HtRHr/1 -> Function Caller/9
  HtRE/1 -> Function Caller/5
  HtRHy/1 -> Function Caller/7
  HtRAr/1 -> Function Caller/17
  HtLE/1 -> Function Caller/6
  HtRAp/1 -> Function Caller/15
  HtLHr/1 -> Function Caller/10
  HtLAp/1 -> Function Caller/16
  HtRSr/1 -> Function Caller/3
  HtRSp/1 -> Function Caller/1
  Function Caller/1 -> com/1
  HtLHy/1 -> Function Caller/8
  HtLAr/1 -> Function Caller/18
  HtLK/1 -> Function Caller/14
  HtLSr/1 -> Function Caller/4
  HtLSp/1 -> Function Caller/2
  HtHp/1 -> Function Caller/20
  Function Caller/2 -> mass/1

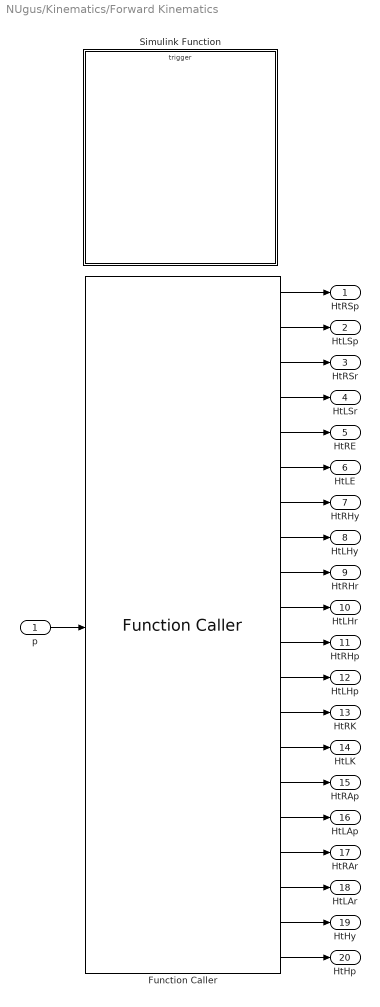
== system NUgus/Kinematics/Forward Kinematics ==
  p : Inport
  Function Caller : FunctionCaller  FunctionPrototype=[HtRSp,HtLSp,HtRSr,HtLSr,HtRE,HtLE,HtRHy,HtLHy,HtRHr,HtLHr,HtRHp,HtLHp,HtRK,HtLK,HtRAp,HtLAp,HtRAr,HtLAr,HtHy,HtHp] = FK(p)  InputArgumentSpecifications=double([1 1 1 1 1 1 1 1 1 1 1 1 1 1 1 1 1 1 1 1])
  Simulink Function : Subsystem  TreatAsAtomicUnit=on
  HtRSp : Outport
  HtLSp : Outport  Port=2
  HtRSr : Outport  Port=3
  HtLSr : Outport  Port=4
  HtRE : Outport  Port=5
  HtLE : Outport  Port=6
  HtRHy : Outport  Port=7
  HtLHy : Outport  Port=8
  HtRHr : Outport  Port=9
  HtLHr : Outport  Port=10
  HtRHp : Outport  Port=11
  HtLHp : Outport  Port=12
  HtRK : Outport  Port=13
  HtLK : Outport  Port=14
  HtRAp : Outport  Port=15
  HtLAp : Outport  Port=16
  HtRAr : Outport  Port=17
  HtLAr : Outport  Port=18
  HtHy : Outport  Port=19
  HtHp : Outport  Port=20
  wires:
  Function Caller/2 -> HtLSp/1
  Function Caller/1 -> HtRSp/1
  Function Caller/3 -> HtRSr/1
  Function Caller/4 -> HtLSr/1
  Function Caller/5 -> HtRE/1
  Function Caller/6 -> HtLE/1
  Function Caller/7 -> HtRHy/1
  Function Caller/8 -> HtLHy/1
  Function Caller/9 -> HtRHr/1
  Function Caller/10 -> HtLHr/1
  Function Caller/11 -> HtRHp/1
  Function Caller/12 -> HtLHp/1
  Function Caller/13 -> HtRK/1
  Function Caller/14 -> HtLK/1
  Function Caller/15 -> HtRAp/1
  Function Caller/16 -> HtLAp/1
  Function Caller/17 -> HtRAr/1
  Function Caller/18 -> HtLAr/1
  Function Caller/19 -> HtHy/1
  Function Caller/20 -> HtHp/1
  p/1 -> Function Caller/1

== system NUgus/Kinematics/Hip Roll Compensation ==
  "hrr_ref " : Inport
  hrl_ref : Inport  Port=2
  theta_ref1 : Inport  Port=3
  theta_ref2 : Inport  Port=4
  Data Store Read : DataStoreRead  Commented=on  DataStoreName=CM740  SampleTime=sample_time  DataStoreElements=CM740.gyro_x
  Inject Control Signal : Subsystem
  Scope : Scope  NumInputPorts=2
  disc to rad/s : Subsystem  Commented=on
  theta_p1 : Outport
  theta_p2 : Outport  Port=2
  wires:
  theta_ref1/1 -> Scope/1, Inject Control Signal/3(theta ref1)
  theta_ref2/1 -> Inject Control Signal/4(theta ref2)
  Data Store Read/1 -> disc to rad/s/1(disc)
  Inject Control Signal/2(theta p2) -> theta_p2/1
  Inject Control Signal/1(theta p1) -> theta_p1/1, Scope/2
  "hrr_ref "/1 -> Inject Control Signal/1(hrr_ref)
  hrl_ref/1 -> Inject Control Signal/2(hrl_ref)

== system NUgus/Kinematics/Hip Roll Compensation1 ==
  "hrr_ref " : Inport
  hrl_ref : Inport  Port=2
  theta_ref1 : Inport  Port=3
  theta_ref2 : Inport  Port=4
  Data Store Read : DataStoreRead  Commented=on  DataStoreName=CM740  SampleTime=sample_time  DataStoreElements=CM740.gyro_x
  Inject Control Signal : Subsystem
  Scope : Scope  NumInputPorts=2
  disc to rad/s : Subsystem  Commented=on
  theta_p1 : Outport
  theta_p2 : Outport  Port=2
  wires:
  theta_ref1/1 -> Scope/1, Inject Control Signal/3(theta ref1)
  theta_ref2/1 -> Inject Control Signal/4(theta ref2)
  Data Store Read/1 -> disc to rad/s/1(disc)
  Inject Control Signal/2(theta p2) -> theta_p2/1
  Inject Control Signal/1(theta p1) -> theta_p1/1, Scope/2
  "hrr_ref "/1 -> Inject Control Signal/1(hrr_ref)
  hrl_ref/1 -> Inject Control Signal/2(hrl_ref)

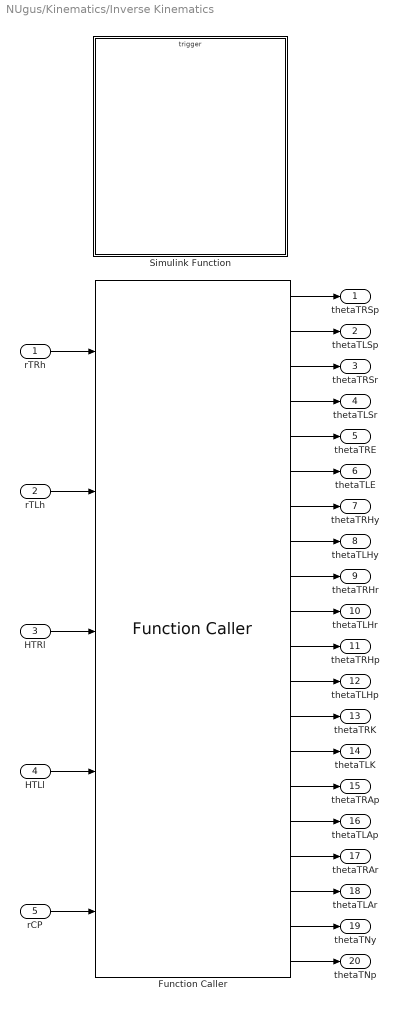
== system NUgus/Kinematics/Inverse Kinematics ==
  rTRh : Inport
  rTLh : Inport  Port=2
  HTRl : Inport  Port=3
  HTLl : Inport  Port=4
  rCP : Inport  Port=5
  Function Caller : FunctionCaller  FunctionPrototype=[thetaTRSp,thetaTLSp,thetaTRSr,thetaTLSr,thetaTRE,thetaTLE,thetaTRHy,thetaTLHy,thetaTRHr,thetaTLHr,thetaTRHp,thetaTLHp,thetaTRK,thetaTLK,thetaTRAp,thetaTLAp,thetaTRAr,thetaTLAr,thetaTNy,thetaTNp] = IK(rTRh,rTLh,HTRl,HTLl,rCP)
  Simulink Function : Subsystem  TreatAsAtomicUnit=on
  thetaTRSp : Outport
  thetaTLSp : Outport  Port=2
  thetaTRSr : Outport  Port=3
  thetaTLSr : Outport  Port=4
  thetaTRE : Outport  Port=5
  thetaTLE : Outport  Port=6
  thetaTRHy : Outport  Port=7
  thetaTLHy : Outport  Port=8
  thetaTRHr : Outport  Port=9
  thetaTLHr : Outport  Port=10
  thetaTRHp : Outport  Port=11
  thetaTLHp : Outport  Port=12
  thetaTRK : Outport  Port=13
  thetaTLK : Outport  Port=14
  thetaTRAp : Outport  Port=15
  thetaTLAp : Outport  Port=16
  thetaTRAr : Outport  Port=17
  thetaTLAr : Outport  Port=18
  thetaTNy : Outport  Port=19
  thetaTNp : Outport  Port=20
  wires:
  Function Caller/2 -> thetaTLSp/1
  Function Caller/1 -> thetaTRSp/1
  Function Caller/3 -> thetaTRSr/1
  Function Caller/4 -> thetaTLSr/1
  Function Caller/5 -> thetaTRE/1
  Function Caller/6 -> thetaTLE/1
  Function Caller/7 -> thetaTRHy/1
  Function Caller/8 -> thetaTLHy/1
  Function Caller/9 -> thetaTRHr/1
  Function Caller/10 -> thetaTLHr/1
  Function Caller/11 -> thetaTRHp/1
  Function Caller/12 -> thetaTLHp/1
  Function Caller/13 -> thetaTRK/1
  Function Caller/14 -> thetaTLK/1
  Function Caller/15 -> thetaTRAp/1
  Function Caller/16 -> thetaTLAp/1
  Function Caller/17 -> thetaTRAr/1
  Function Caller/18 -> thetaTLAr/1
  Function Caller/19 -> thetaTNy/1
  Function Caller/20 -> thetaTNp/1
  rTRh/1 -> Function Caller/1
  rTLh/1 -> Function Caller/2
  HTRl/1 -> Function Caller/3
  HTLl/1 -> Function Caller/4
  rCP/1 -> Function Caller/5

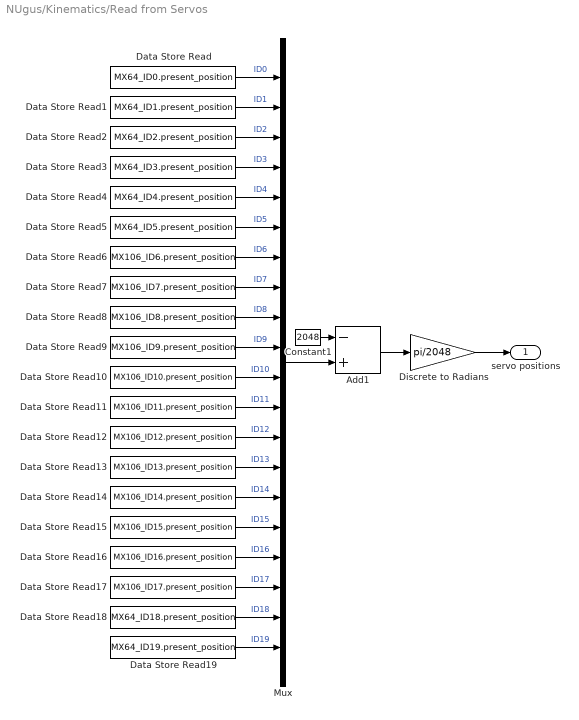
== system NUgus/Kinematics/Read from Servos ==
  Add1 : Sum  Inputs=-+  OutDataTypeStr=double
  Constant1 : Constant  Value=2048
  Data Store Read : DataStoreRead  DataStoreName=MX64_ID0  DataStoreElements=MX64_ID0.present_position
  Data Store Read1 : DataStoreRead  DataStoreName=MX64_ID1  DataStoreElements=MX64_ID1.present_position
  Data Store Read10 : DataStoreRead  DataStoreName=MX106_ID10  DataStoreElements=MX106_ID10.present_position
  Data Store Read11 : DataStoreRead  DataStoreName=MX106_ID11  DataStoreElements=MX106_ID11.present_position
  Data Store Read12 : DataStoreRead  DataStoreName=MX106_ID12  DataStoreElements=MX106_ID12.present_position
  Data Store Read13 : DataStoreRead  DataStoreName=MX106_ID13  DataStoreElements=MX106_ID13.present_position
  Data Store Read14 : DataStoreRead  DataStoreName=MX106_ID14  DataStoreElements=MX106_ID14.present_position
  Data Store Read15 : DataStoreRead  DataStoreName=MX106_ID15  DataStoreElements=MX106_ID15.present_position
  Data Store Read16 : DataStoreRead  DataStoreName=MX106_ID16  DataStoreElements=MX106_ID16.present_position
  Data Store Read17 : DataStoreRead  DataStoreName=MX106_ID17  DataStoreElements=MX106_ID17.present_position
  Data Store Read18 : DataStoreRead  DataStoreName=MX64_ID18  DataStoreElements=MX64_ID18.present_position
  Data Store Read19 : DataStoreRead  DataStoreName=MX64_ID19  DataStoreElements=MX64_ID19.present_position
  Data Store Read2 : DataStoreRead  DataStoreName=MX64_ID2  DataStoreElements=MX64_ID2.present_position
  Data Store Read3 : DataStoreRead  DataStoreName=MX64_ID3  DataStoreElements=MX64_ID3.present_position
  Data Store Read4 : DataStoreRead  DataStoreName=MX64_ID4  DataStoreElements=MX64_ID4.present_position
  Data Store Read5 : DataStoreRead  DataStoreName=MX64_ID5  DataStoreElements=MX64_ID5.present_position
  Data Store Read6 : DataStoreRead  DataStoreName=MX106_ID6  DataStoreElements=MX106_ID6.present_position
  Data Store Read7 : DataStoreRead  DataStoreName=MX106_ID7  DataStoreElements=MX106_ID7.present_position
  Data Store Read8 : DataStoreRead  DataStoreName=MX106_ID8  DataStoreElements=MX106_ID8.present_position
  Data Store Read9 : DataStoreRead  DataStoreName=MX106_ID9  DataStoreElements=MX106_ID9.present_position
  Discrete to Radians : Gain  Gain=pi/2048  SaturateOnIntegerOverflow=on  OutDataTypeStr=Inherit: Same as input
  Mux : Mux  Inputs=20
  servo positions : Outport  PortDimensions=20
  wires:
  Data Store Read19/1 -> Mux/20  "ID19"
  Data Store Read18/1 -> Mux/19  "ID18"
  Data Store Read17/1 -> Mux/18  "ID17"
  Data Store Read/1 -> Mux/1  "ID0"
  Data Store Read1/1 -> Mux/2  "ID1"
  Data Store Read2/1 -> Mux/3  "ID2"
  Data Store Read3/1 -> Mux/4  "ID3"
  Data Store Read4/1 -> Mux/5  "ID4"
  Data Store Read5/1 -> Mux/6  "ID5"
  Data Store Read6/1 -> Mux/7  "ID6"
  Data Store Read7/1 -> Mux/8  "ID7"
  Data Store Read8/1 -> Mux/9  "ID8"
  Data Store Read9/1 -> Mux/10  "ID9"
  Data Store Read10/1 -> Mux/11  "ID10"
  Data Store Read11/1 -> Mux/12  "ID11"
  Data Store Read12/1 -> Mux/13  "ID12"
  Data Store Read13/1 -> Mux/14  "ID13"
  Data Store Read14/1 -> Mux/15  "ID14"
  Data Store Read15/1 -> Mux/16  "ID15"
  Data Store Read16/1 -> Mux/17  "ID16"
  Mux/1 -> Add1/2
  Constant1/1 -> Add1/1
  Add1/1 -> Discrete to Radians/1
  Discrete to Radians/1 -> servo positions/1

== system NUgus/Kinematics/Torso Centre of Mass ==
  HtRSp : Inport
  HtLSp : Inport  Port=2
  HtRSr : Inport  Port=3
  HtLSr : Inport  Port=4
  HtRE : Inport  Port=5
  HtLE : Inport  Port=6
  HtHy : Inport  Port=7
  HtHp : Inport  Port=8
  Function Caller : FunctionCaller  FunctionPrototype=[torso_com,torso_mass] = TorsoCOM(HtRSp,HtLSp,HtRSr,HtLSr,HtRE,HtLE,HtHy,HtHp)
  Simulink Function : Subsystem  TreatAsAtomicUnit=on
  torso_com : Outport
  torso_mass : Outport  Port=2
  wires:
  HtHy/1 -> Function Caller/7
  HtRE/1 -> Function Caller/5
  HtLE/1 -> Function Caller/6
  HtRSr/1 -> Function Caller/3
  HtRSp/1 -> Function Caller/1
  Function Caller/1 -> torso_com/1
  HtLSr/1 -> Function Caller/4
  HtLSp/1 -> Function Caller/2
  HtHp/1 -> Function Caller/8
  Function Caller/2 -> torso_mass/1

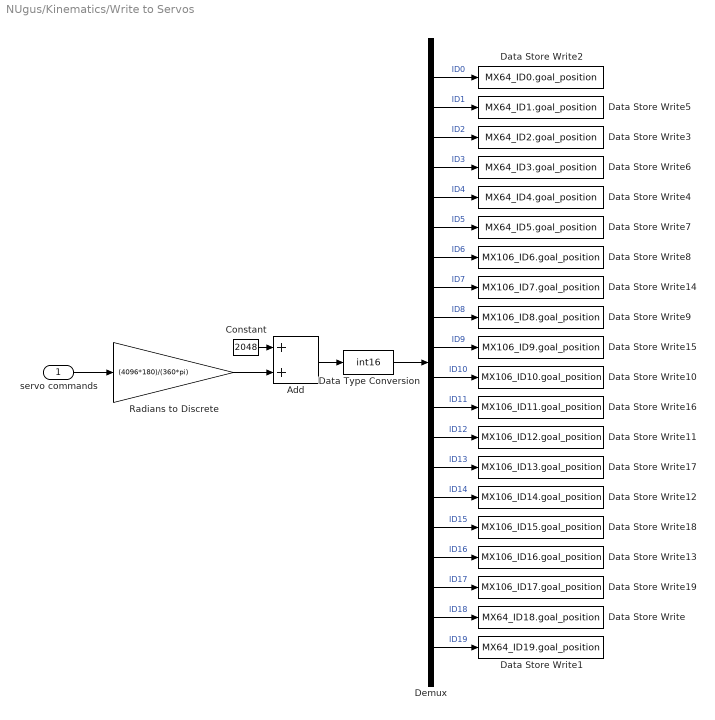
== system NUgus/Kinematics/Write to Servos ==
  servo commands : Inport  PortDimensions=20
  Add : Sum
  Constant : Constant  Value=2048
  Data Store Write : DataStoreWrite  DataStoreName=MX64_ID18  DataStoreElements=MX64_ID18.goal_position
  Data Store Write1 : DataStoreWrite  DataStoreName=MX64_ID19  DataStoreElements=MX64_ID19.goal_position
  Data Store Write10 : DataStoreWrite  DataStoreName=MX106_ID10  DataStoreElements=MX106_ID10.goal_position
  Data Store Write11 : DataStoreWrite  DataStoreName=MX106_ID12  DataStoreElements=MX106_ID12.goal_position
  Data Store Write12 : DataStoreWrite  DataStoreName=MX106_ID14  DataStoreElements=MX106_ID14.goal_position
  Data Store Write13 : DataStoreWrite  DataStoreName=MX106_ID16  DataStoreElements=MX106_ID16.goal_position
  Data Store Write14 : DataStoreWrite  DataStoreName=MX106_ID7  DataStoreElements=MX106_ID7.goal_position
  Data Store Write15 : DataStoreWrite  DataStoreName=MX106_ID9  DataStoreElements=MX106_ID9.goal_position
  Data Store Write16 : DataStoreWrite  DataStoreName=MX106_ID11  DataStoreElements=MX106_ID11.goal_position
  Data Store Write17 : DataStoreWrite  DataStoreName=MX106_ID13  DataStoreElements=MX106_ID13.goal_position
  Data Store Write18 : DataStoreWrite  DataStoreName=MX106_ID15  DataStoreElements=MX106_ID15.goal_position
  Data Store Write19 : DataStoreWrite  DataStoreName=MX106_ID17  DataStoreElements=MX106_ID17.goal_position
  Data Store Write2 : DataStoreWrite  DataStoreName=MX64_ID0  DataStoreElements=MX64_ID0.goal_position
  Data Store Write3 : DataStoreWrite  DataStoreName=MX64_ID2  DataStoreElements=MX64_ID2.goal_position
  Data Store Write4 : DataStoreWrite  DataStoreName=MX64_ID4  DataStoreElements=MX64_ID4.goal_position
  Data Store Write5 : DataStoreWrite  DataStoreName=MX64_ID1  DataStoreElements=MX64_ID1.goal_position
  Data Store Write6 : DataStoreWrite  DataStoreName=MX64_ID3  DataStoreElements=MX64_ID3.goal_position
  Data Store Write7 : DataStoreWrite  DataStoreName=MX64_ID5  DataStoreElements=MX64_ID5.goal_position
  Data Store Write8 : DataStoreWrite  DataStoreName=MX106_ID6  DataStoreElements=MX106_ID6.goal_position
  Data Store Write9 : DataStoreWrite  DataStoreName=MX106_ID8  DataStoreElements=MX106_ID8.goal_position
  Data Type Conversion : DataTypeConversion  OutDataTypeStr=int16
  Demux : Demux  Outputs=20
  Radians to Discrete : Gain  Gain=(4096*180)/(360*pi)  SaturateOnIntegerOverflow=on  OutDataTypeStr=Inherit: Same as input
  wires:
  Demux/3 -> Data Store Write3/1  "ID2"
  Demux/19 -> Data Store Write/1  "ID18"
  Demux/17 -> Data Store Write13/1  "ID16"
  Demux/16 -> Data Store Write18/1  "ID15"
  Demux/6 -> Data Store Write7/1  "ID5"
  Demux/10 -> Data Store Write15/1  "ID9"
  Demux/12 -> Data Store Write16/1  "ID11"
  Demux/20 -> Data Store Write1/1  "ID19"
  Demux/13 -> Data Store Write11/1  "ID12"
  Demux/15 -> Data Store Write12/1  "ID14"
  Demux/18 -> Data Store Write19/1  "ID17"
  Demux/14 -> Data Store Write17/1  "ID13"
  Demux/4 -> Data Store Write6/1  "ID3"
  Demux/1 -> Data Store Write2/1  "ID0"
  Demux/9 -> Data Store Write9/1  "ID8"
  Demux/11 -> Data Store Write10/1  "ID10"
  Demux/2 -> Data Store Write5/1  "ID1"
  Demux/7 -> Data Store Write8/1  "ID6"
  Demux/8 -> Data Store Write14/1  "ID7"
  Demux/5 -> Data Store Write4/1  "ID4"
  Constant/1 -> Add/1
  Radians to Discrete/1 -> Add/2
  Data Type Conversion/1 -> Demux/1
  Add/1 -> Data Type Conversion/1
  servo commands/1 -> Radians to Discrete/1

== system NUgus/Kinematics/to workspace ==
  HtRSp : Inport
  HtLSp : Inport  Port=2
  HtRSr : Inport  Port=3
  HtLSr : Inport  Port=4
  HtRE : Inport  Port=5
  HtLE : Inport  Port=6
  HtRHy : Inport  Port=7
  HtLHy : Inport  Port=8
  HtRHr : Inport  Port=9
  HtLHr : Inport  Port=10
  HtRHp : Inport  Port=11
  HtLHp : Inport  Port=12
  HtRK : Inport  Port=13
  HtLK : Inport  Port=14
  HtRAp : Inport  Port=15
  HtLAp : Inport  Port=16
  HtRAr : Inport  Port=17
  HtLAr : Inport  Port=18
  HtHy : Inport  Port=19
  HtHp : Inport  Port=20
  Bus Creator : BusCreator  Inputs=20
  To Workspace : ToWorkspace  VariableName=FK  SaveFormat=Timeseries  SampleTime=sample_time
  wires:
  HtRHr/1 -> Bus Creator/9
  HtRHp/1 -> Bus Creator/11
  HtRSp/1 -> Bus Creator/1
  HtRHy/1 -> Bus Creator/7
  HtLSr/1 -> Bus Creator/4
  HtLHr/1 -> Bus Creator/10
  Bus Creator/1 -> To Workspace/1
  HtRSr/1 -> Bus Creator/3
  HtRAr/1 -> Bus Creator/17
  HtRE/1 -> Bus Creator/5
  HtLAr/1 -> Bus Creator/18
  HtLHy/1 -> Bus Creator/8
  HtLAp/1 -> Bus Creator/16
  HtLHp/1 -> Bus Creator/12
  HtRAp/1 -> Bus Creator/15
  HtLE/1 -> Bus Creator/6
  HtHp/1 -> Bus Creator/20
  HtRK/1 -> Bus Creator/13
  HtHy/1 -> Bus Creator/19
  HtLK/1 -> Bus Creator/14
  HtLSp/1 -> Bus Creator/2
